simulink model "Energy_Cost"  (Simulink 8.8)
settings: Solver=ode23t  StartTime=0.0  StopTime=24  RelTol=1e-3  EnableMultiTasking=on
model workspace: external: MAT-File (data not in the file)
libraries: simulink x4
(part 3 of 5)

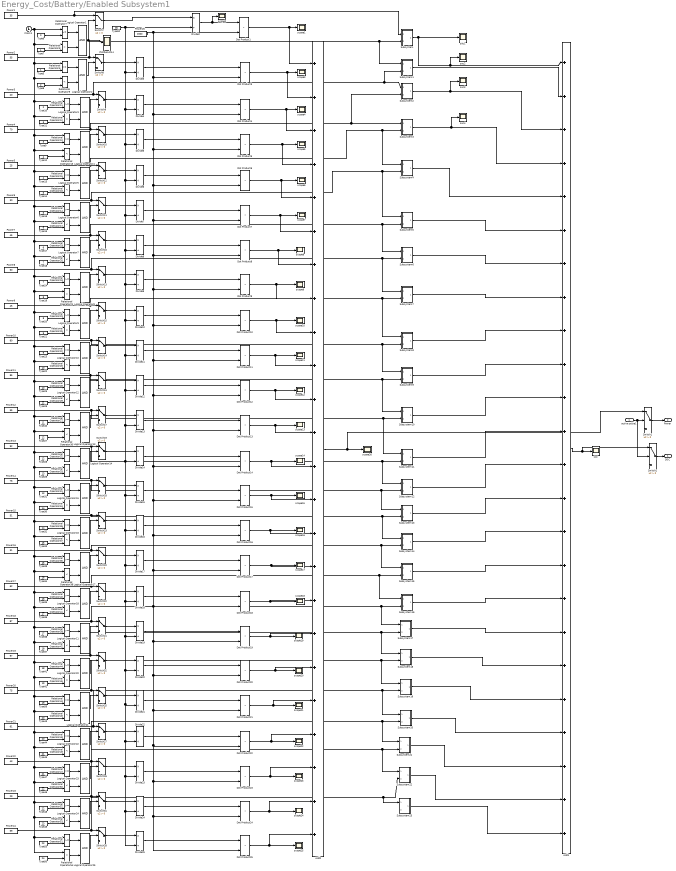
== system Energy_Cost/Battery/Enabled Subsystem1 ==
  active pulse1 : Inport
  Add1 : Sum  Inputs=++++++++++++++++++++++++
  Add2 : Sum  Inputs=++++++++++++++++++++++++
  Clock1 : Clock
  Divide{2..25} (24 alike) : Product  Inputs=*/
  Dot Product{1,3..25} (24 alike) : DotProduct  InputSameDT=on  OutDataTypeStr=Inherit: Inherit via internal rule
  Logical Operator{1..18,20..25} (24 alike) : Logic  AllPortsSameDT=off  OutDataTypeStr=boolean
  PlotResults4 : Scope
  Power1 : Constant  Value=35
  Power10 : Constant  Value=80
  Power11 : Constant  Value=85
  Power12 : Constant  Value=55
  Power13 : Constant  Value=92
  Power14 : Constant  Value=76
  Power15 : Constant  Value=51
  Power16 : Constant  Value=31
  Power17 : Constant  Value=62
  Power18 : Constant  Value=87
  Power19 : Constant  Value=97
  Power2 : Constant  Value=55
  Power20 : Constant  Value=75
  Power21 : Constant  Value=61
  Power22 : Constant  Value=43
  Power23 : Constant  Value=29
  Power24 : Constant  Value=59
  Power25 : Constant  Value=1500
  Power3 : Constant  Value=20
  Power4 : Constant  Value=70
  Power5 : Constant  Value=25
  Power6 : Constant  Value=30
  Power7 : Constant  Value=45
  Power8 : Constant  Value=60
  Power9 : Constant  Value=45
  Relational Operator{6..7,10..11,14..15,18..19,22..23,27..28,31..32,35..36,39..40,43..44,47..48,51..52} (24 alike) : RelationalOperator  RndMeth=Nearest  InputSameDT=on
  Relational Operator{8..9,12..13,16..17,20..21,25..26,29..30,33..34,37..38,41..42,45..46,49..50,53..54} (24 alike) : RelationalOperator  Operator=<  RndMeth=Nearest  InputSameDT=on
  Subsystem : Subsystem
  Subsystem1 : Subsystem
  Subsystem10 : Subsystem
  Subsystem11 : Subsystem
  Subsystem12 : Subsystem
  Subsystem13 : Subsystem
  Subsystem14 : Subsystem
  Subsystem15 : Subsystem
  Subsystem16 : Subsystem
  Subsystem17 : Subsystem
  Subsystem18 : Subsystem
  Subsystem19 : Subsystem
  Subsystem2 : Subsystem
  Subsystem20 : Subsystem
  Subsystem21 : Subsystem
  Subsystem22 : Subsystem
  Subsystem23 : Subsystem
  Subsystem3 : Subsystem
  Subsystem4 : Subsystem
  Subsystem5 : Subsystem
  Subsystem6 : Subsystem
  Subsystem7 : Subsystem
  Subsystem8 : Subsystem
  Subsystem9 : Subsystem
  Switch{1..2,7..28,31..32} (26 alike) : Switch  Criteria=u2 > Threshold
  Type10 : Constant  Value=2
  Type11 : Constant  Value=3
  Type12 : Constant  Value=4
  Type13 : Constant  Value=4
  Type14 : Constant  Value=5
  Type15 : Constant  Value=6
  Type16 : Constant  Value=5
  Type17 : Constant  Value=6
  Type18 : Constant  Value=7
  Type19 : Constant  Value=8
  Type20 : Constant  Value=8
  Type21 : Constant  Value=9
  Type22 : Constant  Value=10
  Type23 : Constant  Value=9
  Type24 : Constant  Value=7
  Type25 : Constant  Value=10
  Type26 : Constant  Value=11
  Type27 : Constant  Value=12
  Type28 : Constant  Value=12
  Type29 : Constant  Value=13
  Type30 : Constant  Value=14
  Type31 : Constant  Value=13
  Type32 : Constant  Value=14
  Type33 : Constant  Value=15
  Type34 : Constant  Value=16
  Type35 : Constant  Value=16
  Type36 : Constant  Value=17
  Type37 : Constant  Value=18
  Type38 : Constant  Value=17
  Type39 : Constant  Value=15
  Type40 : Constant  Value=11
  Type41 : Constant  Value=18
  Type42 : Constant  Value=19
  Type43 : Constant  Value=20
  Type44 : Constant  Value=20
  Type45 : Constant  Value=21
  Type46 : Constant  Value=22
  Type47 : Constant  Value=21
  Type48 : Constant  Value=22
  Type49 : Constant  Value=23
  Type5 : Constant
  Type50 : Constant  Value=24
  Type52 : Constant  Value=35
  Type55 : Constant  Value=23
  Type56 : Constant  Value=19
  Type6 : Constant  Value=0
  Type7 : Constant
  Type8 : Constant  Value=2
  Type9 : Constant  Value=3
  scope{1..26} (26 alike) : Scope
  soc{,1..4} (5 alike) : Scope
  SOC : Outport
  Power : Outport  Port=2
  wires:
  active pulse1/1 -> Switch1/2, Switch2/2
  Type36/1 -> Relational Operator41/2
  Relational Operator41/1 -> Logical Operator18/2
  Type38/1 -> Relational Operator39/2
  Type37/1 -> Relational Operator42/2
  Relational Operator42/1 -> Logical Operator11/2
  Relational Operator39/1 -> Logical Operator11/1
  Logical Operator11/1 -> Switch21/2
  Type41/1 -> Relational Operator44/2
  Type42/1 -> Relational Operator45/2
  Relational Operator45/1 -> Logical Operator20/2
  Relational Operator44/1 -> Logical Operator20/1
  Logical Operator20/1 -> Switch32/2
  Type56/1 -> Relational Operator43/2
  Type43/1 -> Relational Operator46/2
  Relational Operator46/1 -> Logical Operator21/2
  Relational Operator43/1 -> Logical Operator21/1
  Logical Operator21/1 -> Switch25/2
  Type44/1 -> Relational Operator48/2
  Type45/1 -> Relational Operator49/2
  Relational Operator49/1 -> Logical Operator22/2
  Relational Operator48/1 -> Logical Operator22/1
  Logical Operator22/1 -> Switch27/2
  Type47/1 -> Relational Operator47/2
  Type46/1 -> Relational Operator50/2
  Relational Operator50/1 -> Logical Operator23/2
  Relational Operator47/1 -> Logical Operator23/1
  Logical Operator23/1 -> Switch26/2
  Type48/1 -> Relational Operator52/2
  Type49/1 -> Relational Operator53/2
  Relational Operator53/1 -> Logical Operator24/2
  Relational Operator52/1 -> Logical Operator24/1
  Logical Operator24/1 -> Switch31/2
  Type55/1 -> Relational Operator51/2
  Type50/1 -> Relational Operator54/2
  Relational Operator54/1 -> Logical Operator25/2
  Relational Operator51/1 -> Logical Operator25/1
  Logical Operator25/1 -> Switch28/2
  Power18/1 -> Switch21/1, Subsystem16/2(In2), Subsystem17/1(In1)
  Power19/1 -> Switch32/1, Subsystem17/2(In2), Subsystem18/1(In1)
  Power20/1 -> Switch25/1, Subsystem18/2(In2), Subsystem19/1(In1)
  Power21/1 -> Switch27/1, Subsystem19/2(In2), Subsystem20/1(In1)
  Power22/1 -> Switch26/1, Subsystem20/2(In2), Subsystem21/1(In1)
  Power23/1 -> Switch31/1, Subsystem21/2(In2), Subsystem22/1(In1)
  Power24/1 -> Switch28/1, Subsystem22/2(In2), Subsystem23/1(In1)
  Power1/1 -> Switch7/1, Subsystem/1(In1)
  Switch7/1 -> Divide2/1
  Clock1/1 -> Relational Operator7/1, Relational Operator8/1, Relational Operator6/1, Relational Operator9/1, Relational Operator11/1, Relational Operator19/1, Relational Operator20/1, Relational Operator18/1, Relational Operator21/1, Relational Operator23/1, Relational Operator25/1, Relational Operator22/1, Relational Operator26/1, Relational Operator28/1, Relational Operator29/1, Relational Operator27/1, Relational Operator32/1, Relational Operator31/1, Relational Operator34/1, Relational Operator36/1, Relational Operator37/1, Relational Operator35/1, Relational Operator38/1, Relational Operator40/1, Relational Operator41/1, Relational Operator39/1, Relational Operator42/1, Relational Operator45/1, Relational Operator43/1, Relational Operator47/1, Relational Operator54/1, Relational Operator51/1, Relational Operator53/1, Relational Operator52/1, Relational Operator50/1, Relational Operator49/1, Relational Operator48/1, Relational Operator46/1, Relational Operator44/1, Relational Operator33/1, Relational Operator30/1, Relational Operator17/1, Relational Operator14/1, Relational Operator16/1, Relational Operator15/1, Relational Operator13/1, Relational Operator10/1, Relational Operator12/1
  Type6/1 -> Relational Operator7/2
  Relational Operator7/1 -> Logical Operator1/1
  Power2/1 -> Switch8/1, Subsystem/2(In2), Subsystem1/1(In1)
  Type5/1 -> Relational Operator6/2
  Relational Operator6/1 -> Logical Operator2/1
  Type10/1 -> Relational Operator11/2
  Relational Operator11/1 -> Logical Operator3/1
  Type9/1 -> Relational Operator10/2
  Type12/1 -> Relational Operator13/2
  Relational Operator13/1 -> Logical Operator4/2
  Relational Operator10/1 -> Logical Operator4/1
  Logical Operator4/1 -> Switch10/2
  Type13/1 -> Relational Operator15/2
  Type14/1 -> Relational Operator16/2
  Relational Operator16/1 -> Logical Operator5/2
  Relational Operator15/1 -> Logical Operator5/1
  Logical Operator5/1 -> Switch12/2
  Type16/1 -> Relational Operator14/2
  Type15/1 -> Relational Operator17/2
  Relational Operator17/1 -> Logical Operator6/2
  Relational Operator14/1 -> Logical Operator6/1
  Logical Operator6/1 -> Switch11/2
  Type17/1 -> Relational Operator19/2
  Type18/1 -> Relational Operator20/2
  Relational Operator20/1 -> Logical Operator7/2
  Relational Operator19/1 -> Logical Operator7/1
  Logical Operator7/1 -> Switch16/2
  Type24/1 -> Relational Operator18/2
  Type19/1 -> Relational Operator21/2
  Relational Operator21/1 -> Logical Operator8/2
  Relational Operator18/1 -> Logical Operator8/1
  Logical Operator8/1 -> Switch13/2
  Type20/1 -> Relational Operator23/2
  Type21/1 -> Relational Operator25/2
  Relational Operator25/1 -> Logical Operator9/2
  Relational Operator23/1 -> Logical Operator9/1
  Logical Operator9/1 -> Switch15/2
  Type23/1 -> Relational Operator22/2
  Type22/1 -> Relational Operator26/2
  Relational Operator26/1 -> Logical Operator10/2
  Relational Operator22/1 -> Logical Operator10/1
  Logical Operator10/1 -> Switch14/2
  Type25/1 -> Relational Operator28/2
  Type26/1 -> Relational Operator29/2
  Relational Operator29/1 -> Logical Operator12/2
  Relational Operator28/1 -> Logical Operator12/1
  Logical Operator12/1 -> Switch24/2
  Type40/1 -> Relational Operator27/2
  Type27/1 -> Relational Operator30/2
  Relational Operator30/1 -> Logical Operator13/2
  Relational Operator27/1 -> Logical Operator13/1
  Logical Operator13/1 -> Switch17/2
  Type28/1 -> Relational Operator32/2
  Type29/1 -> Relational Operator33/2
  Relational Operator33/1 -> Logical Operator14/2
  Relational Operator32/1 -> Logical Operator14/1
  Logical Operator14/1 -> Switch19/2
  Type31/1 -> Relational Operator31/2
  Type30/1 -> Relational Operator34/2
  Relational Operator34/1 -> Logical Operator15/2
  Relational Operator31/1 -> Logical Operator15/1
  Logical Operator15/1 -> Switch18/2
  Type32/1 -> Relational Operator36/2
  Type33/1 -> Relational Operator37/2
  Relational Operator37/1 -> Logical Operator16/2
  Relational Operator36/1 -> Logical Operator16/1
  Logical Operator16/1 -> Switch23/2
  Type39/1 -> Relational Operator35/2
  Type34/1 -> Relational Operator38/2
  Relational Operator38/1 -> Logical Operator17/2
  Relational Operator35/1 -> Logical Operator17/1
  Logical Operator17/1 -> Switch20/2
  Type35/1 -> Relational Operator40/2
  Relational Operator40/1 -> Logical Operator18/1
  Logical Operator18/1 -> Switch22/2
  Power3/1 -> Switch9/1, Subsystem1/2(In2), Subsystem2/1(In1)
  Power4/1 -> Switch10/1, Subsystem2/2(In2), Subsystem3/1(In1)
  Power5/1 -> Switch12/1, Subsystem3/2(In2), Subsystem4/1(In1)
  Power6/1 -> Switch11/1, Subsystem4/2(In2), Subsystem5/1(In1)
  Power7/1 -> Switch16/1, Subsystem5/2(In2), Subsystem6/1(In1)
  Power8/1 -> Switch13/1, Subsystem6/2(In2), Subsystem7/1(In1)
  Power9/1 -> Switch15/1, Subsystem7/2(In2), Subsystem8/1(In1)
  Power10/1 -> Switch14/1, Subsystem8/2(In2), Subsystem9/1(In1)
  Power11/1 -> Switch24/1, Subsystem9/2(In2), Subsystem10/1(In1)
  Power12/1 -> Switch17/1, Subsystem10/2(In2), Subsystem11/1(In1)
  Power13/1 -> Switch19/1, Subsystem11/2(In2), Subsystem12/1(In1)
  Power14/1 -> Switch18/1, Subsystem12/2(In2), Subsystem13/1(In1)
  Power15/1 -> Switch23/1, Subsystem13/2(In2), Subsystem14/1(In1)
  Power16/1 -> Switch20/1, Subsystem14/2(In2), Subsystem15/1(In1)
  Power17/1 -> Switch22/1, Subsystem15/2(In2), Subsystem16/1(In1)
  Type52/1 -> Divide2/2, Divide3/2, Divide4/2, Divide5/2, Divide9/2, Divide10/2, Divide12/2, Divide13/2, Divide18/2, Divide19/2, Divide20/2, Divide21/2, Divide22/2, Divide23/2, Divide25/2, Divide24/2, Divide17/2, Divide16/2, Divide15/2, Divide14/2, Divide11/2, Divide8/2, Divide7/2, Divide6/2
  Divide2/1 -> Dot Product1/1, scope2/1
  Power25/1 -> Dot Product1/2, Dot Product3/2, Dot Product4/2, Dot Product6/2, Dot Product7/2, Dot Product12/2, Dot Product13/2, Dot Product14/2, Dot Product18/2, Dot Product19/2, Dot Product20/2, Dot Product21/2, Dot Product22/2, Dot Product23/2, Dot Product25/2, Dot Product24/2, Dot Product17/2, Dot Product16/2, Dot Product15/2, Dot Product11/2, Dot Product10/2, Dot Product9/2, Dot Product8/2, Dot Product5/2
  Dot Product1/1 -> scope1/1, Add2/1
  Switch8/1 -> Divide3/1
  Divide3/1 -> Dot Product3/1
  Dot Product3/1 -> scope3/1, Add2/2
  Divide4/1 -> Dot Product4/1
  Dot Product4/1 -> scope4/1, Add2/3
  Divide5/1 -> Dot Product5/1
  Dot Product5/1 -> scope5/1, Add2/4
  Divide6/1 -> Dot Product6/1
  Dot Product6/1 -> scope6/1, Add2/5
  Divide7/1 -> Dot Product7/1
  Dot Product7/1 -> scope7/1, Add2/6
  Divide8/1 -> Dot Product8/1
  Dot Product8/1 -> scope8/1, Add2/7
  Divide9/1 -> Dot Product9/1
  Dot Product9/1 -> scope9/1, Add2/8
  Divide10/1 -> Dot Product10/1
  Dot Product10/1 -> scope10/1, Add2/9
  Divide11/1 -> Dot Product11/1
  Dot Product11/1 -> scope11/1, Add2/10
  Divide12/1 -> Dot Product12/1
  Dot Product12/1 -> scope12/1, Add2/11
  Divide13/1 -> Dot Product13/1
  Dot Product13/1 -> scope13/1, Add2/12
  Divide14/1 -> Dot Product14/1
  Dot Product14/1 -> scope14/1, Add2/13
  Divide15/1 -> Dot Product15/1
  Dot Product15/1 -> scope15/1, Add2/14
  Divide16/1 -> Dot Product16/1
  Dot Product16/1 -> scope16/1, Add2/15
  Divide17/1 -> Dot Product17/1
  Dot Product17/1 -> scope17/1, Add2/16
  Divide18/1 -> Dot Product18/1
  Dot Product18/1 -> scope18/1, Add2/17
  Divide19/1 -> Dot Product19/1
  Dot Product19/1 -> scope19/1, Add2/18
  Divide20/1 -> Dot Product20/1
  Dot Product20/1 -> scope20/1, Add2/19
  Divide21/1 -> Dot Product21/1
  Dot Product21/1 -> scope21/1, Add2/20
  Divide22/1 -> Dot Product22/1
  Dot Product22/1 -> scope22/1, Add2/21
  Divide23/1 -> Dot Product23/1
  Dot Product23/1 -> scope23/1, Add2/22
  Divide24/1 -> Dot Product24/1
  Dot Product24/1 -> scope24/1, Add2/23
  Divide25/1 -> Dot Product25/1
  Dot Product25/1 -> scope25/1, Add2/24
  Switch28/1 -> Divide25/1
  Switch31/1 -> Divide24/1
  Switch26/1 -> Divide23/1
  Switch27/1 -> Divide22/1
  Switch25/1 -> Divide21/1
  Switch32/1 -> Divide20/1
  Switch21/1 -> Divide19/1
  Switch22/1 -> Divide18/1
  Switch20/1 -> Divide17/1
  Switch23/1 -> Divide16/1
  Switch18/1 -> Divide15/1
  Switch19/1 -> Divide14/1
  Switch17/1 -> Divide13/1
  Switch24/1 -> Divide12/1
  Switch14/1 -> Divide11/1
  Switch15/1 -> Divide10/1
  Switch13/1 -> Divide9/1
  Switch16/1 -> Divide8/1
  Switch11/1 -> Divide7/1
  Switch12/1 -> Divide6/1
  Switch10/1 -> Divide5/1
  Switch9/1 -> Divide4/1
  Add2/1 -> scope26/1, Switch1/1
  Logical Operator3/1 -> Switch9/2
  Relational Operator12/1 -> Logical Operator3/2
  Type11/1 -> Relational Operator12/2
  Logical Operator2/1 -> Switch8/2
  Type8/1 -> Relational Operator9/2
  Relational Operator9/1 -> Logical Operator2/2
  Logical Operator1/1 -> Switch7/2, PlotResults4/1
  Type7/1 -> Relational Operator8/2
  Relational Operator8/1 -> Logical Operator1/2
  Subsystem/1(Out1) -> soc1/1, Add1/1, soc2/1
  Subsystem1/1(Out1) -> Add1/2
  Subsystem2/1(Out1) -> soc3/1, Add1/3
  Subsystem3/1(Out1) -> Add1/4, soc4/1
  Add1/1 -> soc/1, Switch2/1
  Subsystem4/1(Out1) -> Add1/5
  Subsystem5/1(Out1) -> Add1/6
  Subsystem6/1(Out1) -> Add1/7
  Subsystem7/1(Out1) -> Add1/8
  Subsystem8/1(Out1) -> Add1/9
  Subsystem9/1(Out1) -> Add1/10
  Subsystem10/1(Out1) -> Add1/11
  Subsystem11/1(Out1) -> Add1/12
  Subsystem12/1(Out1) -> Add1/13
  Subsystem13/1(Out1) -> Add1/14
  Subsystem14/1(Out1) -> Add1/15
  Subsystem15/1(Out1) -> Add1/16
  Subsystem16/1(Out1) -> Add1/17
  Subsystem17/1(Out1) -> Add1/18
  Subsystem18/1(Out1) -> Add1/19
  Subsystem19/1(Out1) -> Add1/20
  Subsystem20/1(Out1) -> Add1/21
  Subsystem21/1(Out1) -> Add1/22
  Subsystem22/1(Out1) -> Add1/23
  Subsystem23/1(Out1) -> Add1/24
  Switch2/1 -> SOC/1
  Switch1/1 -> Power/1

== system Energy_Cost/Battery/Rates ==
  Powe_cons : Inport
  Rate_season : Inport  Port=2
  Clock1 : Clock
      settings: Decimation=100
  Constant : Constant  Value=6.2
  Constant1 : Constant  Value=10.8
  Constant2 : Constant  Value=9.2
  Electricity Rate : M-S-Function  FunctionName=Elec_Rate_Fun
  Heater Switch1 : Product  RndMeth=Zero
  Rate : Outport  InitialOutput=0
  wires:
  Rate_season/1 -> Electricity Rate/5
  Clock1/1 -> Electricity Rate/4
  Constant/1 -> Electricity Rate/1
  Heater Switch1/1 -> Rate/1
  Powe_cons/1 -> Heater Switch1/2
  Electricity Rate/1 -> Heater Switch1/1  "Elec_Rate"
  Constant1/1 -> Electricity Rate/3
  Constant2/1 -> Electricity Rate/2

== system Energy_Cost/Battery/Subsystem ==
  In1 : Inport
  In2 : Inport  Port=2
  Clock2 : Clock
  Divide26 : Product  Inputs=*/
  Dot Product2 : DotProduct  InputSameDT=on  OutDataTypeStr=Inherit: Inherit via internal rule
  Logical Operator19 : Logic  AllPortsSameDT=off  OutDataTypeStr=boolean
  Relational Operator2 : RelationalOperator  RndMeth=Nearest  InputSameDT=on
  Relational Operator3 : RelationalOperator  Operator=<  RndMeth=Nearest  InputSameDT=on
  Sum : Sum  Inputs=|++
  Sum1 : Sum  Inputs=|-+
  Switch2 : Switch  Criteria=u2 > Threshold
  Type54 : Constant
  Type57 : Constant  Value=0
  Type58 : Constant
  soc3 : Scope
  Out1 : Outport
  wires:
  Sum1/1 -> Divide26/1
  Type54/1 -> Divide26/2
  Divide26/1 -> Dot Product2/1
  Clock2/1 -> Dot Product2/2, Relational Operator3/1, Relational Operator2/1
  Dot Product2/1 -> Sum/2
  Sum/1 -> Switch2/1
  Type57/1 -> Relational Operator2/2
  Relational Operator2/1 -> Logical Operator19/1
  Type58/1 -> Relational Operator3/2
  Relational Operator3/1 -> Logical Operator19/2
  Logical Operator19/1 -> Switch2/2
  In1/1 -> Sum/1, Sum1/1
  In2/1 -> Sum1/2
  Switch2/1 -> Out1/1, soc3/1

== system Energy_Cost/Battery/Subsystem1 ==
  In1 : Inport
  In2 : Inport  Port=2
  Clock2 : Clock
  Divide26 : Product  Inputs=*/
  Dot Product2 : DotProduct  InputSameDT=on  OutDataTypeStr=Inherit: Inherit via internal rule
  Logical Operator19 : Logic  AllPortsSameDT=off  OutDataTypeStr=boolean
  Relational Operator2 : RelationalOperator  RndMeth=Nearest  InputSameDT=on
  Relational Operator3 : RelationalOperator  Operator=<  RndMeth=Nearest  InputSameDT=on
  Sum : Sum  Inputs=|++
  Sum1 : Sum  Inputs=|-+
  Sum2 : Sum  Inputs=|+-
  Switch2 : Switch  Criteria=u2 > Threshold
  Type1 : Constant
  Type54 : Constant
  Type57 : Constant
  Type58 : Constant  Value=2
  soc1 : Scope
  Out1 : Outport
  wires:
  Switch2/1 -> Out1/1, soc1/1
  In2/1 -> Sum1/2
  In1/1 -> Sum1/1, Sum/1
  Logical Operator19/1 -> Switch2/2
  Relational Operator3/1 -> Logical Operator19/2
  Type58/1 -> Relational Operator3/2
  Relational Operator2/1 -> Logical Operator19/1
  Type57/1 -> Relational Operator2/2
  Sum/1 -> Switch2/1
  Dot Product2/1 -> Sum/2
  Divide26/1 -> Dot Product2/1
  Type54/1 -> Divide26/2
  Sum1/1 -> Divide26/1
  Clock2/1 -> Sum2/1, Relational Operator2/1, Relational Operator3/1
  Type1/1 -> Sum2/2
  Sum2/1 -> Dot Product2/2

== system Energy_Cost/Battery/Subsystem10 ==
  In1 : Inport
  In2 : Inport  Port=2
  Clock2 : Clock
  Divide26 : Product  Inputs=*/
  Dot Product2 : DotProduct  InputSameDT=on  OutDataTypeStr=Inherit: Inherit via internal rule
  Logical Operator19 : Logic  AllPortsSameDT=off  OutDataTypeStr=boolean
  Relational Operator2 : RelationalOperator  RndMeth=Nearest  InputSameDT=on
  Relational Operator3 : RelationalOperator  Operator=<  RndMeth=Nearest  InputSameDT=on
  Sum : Sum  Inputs=|++
  Sum1 : Sum  Inputs=|-+
  Sum2 : Sum  Inputs=|+-
  Switch2 : Switch  Criteria=u2 > Threshold
  Type1 : Constant  Value=10
  Type54 : Constant
  Type57 : Constant  Value=10
  Type58 : Constant  Value=11
  soc1 : Scope
  Out1 : Outport
  wires:
  Sum2/1 -> Dot Product2/2
  Type1/1 -> Sum2/2
  Clock2/1 -> Relational Operator3/1, Relational Operator2/1, Sum2/1
  Sum1/1 -> Divide26/1
  Type54/1 -> Divide26/2
  Divide26/1 -> Dot Product2/1
  Dot Product2/1 -> Sum/2
  Sum/1 -> Switch2/1
  Type57/1 -> Relational Operator2/2
  Relational Operator2/1 -> Logical Operator19/1
  Type58/1 -> Relational Operator3/2
  Relational Operator3/1 -> Logical Operator19/2
  Logical Operator19/1 -> Switch2/2
  In1/1 -> Sum/1, Sum1/1
  In2/1 -> Sum1/2
  Switch2/1 -> soc1/1, Out1/1

== system Energy_Cost/Battery/Subsystem11 ==
  In1 : Inport
  In2 : Inport  Port=2
  Clock2 : Clock
  Divide26 : Product  Inputs=*/
  Dot Product2 : DotProduct  InputSameDT=on  OutDataTypeStr=Inherit: Inherit via internal rule
  Logical Operator19 : Logic  AllPortsSameDT=off  OutDataTypeStr=boolean
  Relational Operator2 : RelationalOperator  RndMeth=Nearest  InputSameDT=on
  Relational Operator3 : RelationalOperator  Operator=<  RndMeth=Nearest  InputSameDT=on
  Sum : Sum  Inputs=|++
  Sum1 : Sum  Inputs=|-+
  Sum2 : Sum  Inputs=|+-
  Switch2 : Switch  Criteria=u2 > Threshold
  Type1 : Constant  Value=11
  Type54 : Constant
  Type57 : Constant  Value=11
  Type58 : Constant  Value=12
  soc1 : Scope
  Out1 : Outport
  wires:
  Switch2/1 -> Out1/1, soc1/1
  In2/1 -> Sum1/2
  In1/1 -> Sum1/1, Sum/1
  Logical Operator19/1 -> Switch2/2
  Relational Operator3/1 -> Logical Operator19/2
  Type58/1 -> Relational Operator3/2
  Relational Operator2/1 -> Logical Operator19/1
  Type57/1 -> Relational Operator2/2
  Sum/1 -> Switch2/1
  Dot Product2/1 -> Sum/2
  Divide26/1 -> Dot Product2/1
  Type54/1 -> Divide26/2
  Sum1/1 -> Divide26/1
  Clock2/1 -> Sum2/1, Relational Operator2/1, Relational Operator3/1
  Type1/1 -> Sum2/2
  Sum2/1 -> Dot Product2/2

== system Energy_Cost/Battery/Subsystem12 ==
  In1 : Inport
  In2 : Inport  Port=2
  Clock2 : Clock
  Divide26 : Product  Inputs=*/
  Dot Product2 : DotProduct  InputSameDT=on  OutDataTypeStr=Inherit: Inherit via internal rule
  Logical Operator19 : Logic  AllPortsSameDT=off  OutDataTypeStr=boolean
  Relational Operator2 : RelationalOperator  RndMeth=Nearest  InputSameDT=on
  Relational Operator3 : RelationalOperator  Operator=<  RndMeth=Nearest  InputSameDT=on
  Sum : Sum  Inputs=|++
  Sum1 : Sum  Inputs=|-+
  Sum2 : Sum  Inputs=|+-
  Switch2 : Switch  Criteria=u2 > Threshold
  Type1 : Constant  Value=12
  Type54 : Constant
  Type57 : Constant  Value=12
  Type58 : Constant  Value=13
  soc1 : Scope
  Out1 : Outport
  wires:
  Sum2/1 -> Dot Product2/2
  Type1/1 -> Sum2/2
  Clock2/1 -> Relational Operator3/1, Relational Operator2/1, Sum2/1
  Sum1/1 -> Divide26/1
  Type54/1 -> Divide26/2
  Divide26/1 -> Dot Product2/1
  Dot Product2/1 -> Sum/2
  Sum/1 -> Switch2/1
  Type57/1 -> Relational Operator2/2
  Relational Operator2/1 -> Logical Operator19/1
  Type58/1 -> Relational Operator3/2
  Relational Operator3/1 -> Logical Operator19/2
  Logical Operator19/1 -> Switch2/2
  In1/1 -> Sum/1, Sum1/1
  In2/1 -> Sum1/2
  Switch2/1 -> soc1/1, Out1/1

== system Energy_Cost/Battery/Subsystem13 ==
  In1 : Inport
  In2 : Inport  Port=2
  Clock2 : Clock
  Divide26 : Product  Inputs=*/
  Dot Product2 : DotProduct  InputSameDT=on  OutDataTypeStr=Inherit: Inherit via internal rule
  Logical Operator19 : Logic  AllPortsSameDT=off  OutDataTypeStr=boolean
  Relational Operator2 : RelationalOperator  RndMeth=Nearest  InputSameDT=on
  Relational Operator3 : RelationalOperator  Operator=<  RndMeth=Nearest  InputSameDT=on
  Sum : Sum  Inputs=|++
  Sum1 : Sum  Inputs=|-+
  Sum2 : Sum  Inputs=|+-
  Switch2 : Switch  Criteria=u2 > Threshold
  Type1 : Constant  Value=13
  Type54 : Constant
  Type57 : Constant  Value=13
  Type58 : Constant  Value=14
  soc1 : Scope
  Out1 : Outport
  wires:
  Switch2/1 -> Out1/1, soc1/1
  In2/1 -> Sum1/2
  In1/1 -> Sum1/1, Sum/1
  Logical Operator19/1 -> Switch2/2
  Relational Operator3/1 -> Logical Operator19/2
  Type58/1 -> Relational Operator3/2
  Relational Operator2/1 -> Logical Operator19/1
  Type57/1 -> Relational Operator2/2
  Sum/1 -> Switch2/1
  Dot Product2/1 -> Sum/2
  Divide26/1 -> Dot Product2/1
  Type54/1 -> Divide26/2
  Sum1/1 -> Divide26/1
  Clock2/1 -> Sum2/1, Relational Operator2/1, Relational Operator3/1
  Type1/1 -> Sum2/2
  Sum2/1 -> Dot Product2/2

== system Energy_Cost/Battery/Subsystem14 ==
  In1 : Inport
  In2 : Inport  Port=2
  Clock2 : Clock
  Divide26 : Product  Inputs=*/
  Dot Product2 : DotProduct  InputSameDT=on  OutDataTypeStr=Inherit: Inherit via internal rule
  Logical Operator19 : Logic  AllPortsSameDT=off  OutDataTypeStr=boolean
  Relational Operator2 : RelationalOperator  RndMeth=Nearest  InputSameDT=on
  Relational Operator3 : RelationalOperator  Operator=<  RndMeth=Nearest  InputSameDT=on
  Sum : Sum  Inputs=|++
  Sum1 : Sum  Inputs=|-+
  Sum2 : Sum  Inputs=|+-
  Switch2 : Switch  Criteria=u2 > Threshold
  Type1 : Constant  Value=14
  Type54 : Constant
  Type57 : Constant  Value=14
  Type58 : Constant  Value=15
  soc1 : Scope
  Out1 : Outport
  wires:
  Sum2/1 -> Dot Product2/2
  Type1/1 -> Sum2/2
  Clock2/1 -> Relational Operator3/1, Relational Operator2/1, Sum2/1
  Sum1/1 -> Divide26/1
  Type54/1 -> Divide26/2
  Divide26/1 -> Dot Product2/1
  Dot Product2/1 -> Sum/2
  Sum/1 -> Switch2/1
  Type57/1 -> Relational Operator2/2
  Relational Operator2/1 -> Logical Operator19/1
  Type58/1 -> Relational Operator3/2
  Relational Operator3/1 -> Logical Operator19/2
  Logical Operator19/1 -> Switch2/2
  In1/1 -> Sum/1, Sum1/1
  In2/1 -> Sum1/2
  Switch2/1 -> soc1/1, Out1/1

== system Energy_Cost/Battery/Subsystem15 ==
  In1 : Inport
  In2 : Inport  Port=2
  Clock2 : Clock
  Divide26 : Product  Inputs=*/
  Dot Product2 : DotProduct  InputSameDT=on  OutDataTypeStr=Inherit: Inherit via internal rule
  Logical Operator19 : Logic  AllPortsSameDT=off  OutDataTypeStr=boolean
  Relational Operator2 : RelationalOperator  RndMeth=Nearest  InputSameDT=on
  Relational Operator3 : RelationalOperator  Operator=<  RndMeth=Nearest  InputSameDT=on
  Sum : Sum  Inputs=|++
  Sum1 : Sum  Inputs=|-+
  Sum2 : Sum  Inputs=|+-
  Switch2 : Switch  Criteria=u2 > Threshold
  Type1 : Constant  Value=15
  Type54 : Constant
  Type57 : Constant  Value=15
  Type58 : Constant  Value=16
  soc1 : Scope
  Out1 : Outport
  wires:
  Switch2/1 -> Out1/1, soc1/1
  In2/1 -> Sum1/2
  In1/1 -> Sum1/1, Sum/1
  Logical Operator19/1 -> Switch2/2
  Relational Operator3/1 -> Logical Operator19/2
  Type58/1 -> Relational Operator3/2
  Relational Operator2/1 -> Logical Operator19/1
  Type57/1 -> Relational Operator2/2
  Sum/1 -> Switch2/1
  Dot Product2/1 -> Sum/2
  Divide26/1 -> Dot Product2/1
  Type54/1 -> Divide26/2
  Sum1/1 -> Divide26/1
  Clock2/1 -> Sum2/1, Relational Operator2/1, Relational Operator3/1
  Type1/1 -> Sum2/2
  Sum2/1 -> Dot Product2/2

== system Energy_Cost/Battery/Subsystem16 ==
  In1 : Inport
  In2 : Inport  Port=2
  Clock2 : Clock
  Divide26 : Product  Inputs=*/
  Dot Product2 : DotProduct  InputSameDT=on  OutDataTypeStr=Inherit: Inherit via internal rule
  Logical Operator19 : Logic  AllPortsSameDT=off  OutDataTypeStr=boolean
  Relational Operator2 : RelationalOperator  RndMeth=Nearest  InputSameDT=on
  Relational Operator3 : RelationalOperator  Operator=<  RndMeth=Nearest  InputSameDT=on
  Sum : Sum  Inputs=|++
  Sum1 : Sum  Inputs=|-+
  Sum2 : Sum  Inputs=|+-
  Switch2 : Switch  Criteria=u2 > Threshold
  Type1 : Constant  Value=16
  Type54 : Constant
  Type57 : Constant  Value=16
  Type58 : Constant  Value=17
  soc1 : Scope
  Out1 : Outport
  wires:
  Sum2/1 -> Dot Product2/2
  Type1/1 -> Sum2/2
  Clock2/1 -> Relational Operator3/1, Relational Operator2/1, Sum2/1
  Sum1/1 -> Divide26/1
  Type54/1 -> Divide26/2
  Divide26/1 -> Dot Product2/1
  Dot Product2/1 -> Sum/2
  Sum/1 -> Switch2/1
  Type57/1 -> Relational Operator2/2
  Relational Operator2/1 -> Logical Operator19/1
  Type58/1 -> Relational Operator3/2
  Relational Operator3/1 -> Logical Operator19/2
  Logical Operator19/1 -> Switch2/2
  In1/1 -> Sum/1, Sum1/1
  In2/1 -> Sum1/2
  Switch2/1 -> soc1/1, Out1/1

== system Energy_Cost/Battery/Subsystem17 ==
  In1 : Inport
  In2 : Inport  Port=2
  Clock2 : Clock
  Divide26 : Product  Inputs=*/
  Dot Product2 : DotProduct  InputSameDT=on  OutDataTypeStr=Inherit: Inherit via internal rule
  Logical Operator19 : Logic  AllPortsSameDT=off  OutDataTypeStr=boolean
  Relational Operator2 : RelationalOperator  RndMeth=Nearest  InputSameDT=on
  Relational Operator3 : RelationalOperator  Operator=<  RndMeth=Nearest  InputSameDT=on
  Sum : Sum  Inputs=|++
  Sum1 : Sum  Inputs=|-+
  Sum2 : Sum  Inputs=|+-
  Switch2 : Switch  Criteria=u2 > Threshold
  Type1 : Constant  Value=17
  Type54 : Constant
  Type57 : Constant  Value=17
  Type58 : Constant  Value=18
  soc1 : Scope
  Out1 : Outport
  wires:
  Sum2/1 -> Dot Product2/2
  Type1/1 -> Sum2/2
  Clock2/1 -> Relational Operator3/1, Relational Operator2/1, Sum2/1
  Sum1/1 -> Divide26/1
  Type54/1 -> Divide26/2
  Divide26/1 -> Dot Product2/1
  Dot Product2/1 -> Sum/2
  Sum/1 -> Switch2/1
  Type57/1 -> Relational Operator2/2
  Relational Operator2/1 -> Logical Operator19/1
  Type58/1 -> Relational Operator3/2
  Relational Operator3/1 -> Logical Operator19/2
  Logical Operator19/1 -> Switch2/2
  In1/1 -> Sum/1, Sum1/1
  In2/1 -> Sum1/2
  Switch2/1 -> soc1/1, Out1/1

== system Energy_Cost/Battery/Subsystem18 ==
  In1 : Inport
  In2 : Inport  Port=2
  Clock2 : Clock
  Divide26 : Product  Inputs=*/
  Dot Product2 : DotProduct  InputSameDT=on  OutDataTypeStr=Inherit: Inherit via internal rule
  Logical Operator19 : Logic  AllPortsSameDT=off  OutDataTypeStr=boolean
  Relational Operator2 : RelationalOperator  RndMeth=Nearest  InputSameDT=on
  Relational Operator3 : RelationalOperator  Operator=<  RndMeth=Nearest  InputSameDT=on
  Sum : Sum  Inputs=|++
  Sum1 : Sum  Inputs=|-+
  Sum2 : Sum  Inputs=|+-
  Switch2 : Switch  Criteria=u2 > Threshold
  Type1 : Constant  Value=18
  Type54 : Constant
  Type57 : Constant  Value=18
  Type58 : Constant  Value=19
  soc1 : Scope
  Out1 : Outport
  wires:
  Switch2/1 -> Out1/1, soc1/1
  In2/1 -> Sum1/2
  In1/1 -> Sum1/1, Sum/1
  Logical Operator19/1 -> Switch2/2
  Relational Operator3/1 -> Logical Operator19/2
  Type58/1 -> Relational Operator3/2
  Relational Operator2/1 -> Logical Operator19/1
  Type57/1 -> Relational Operator2/2
  Sum/1 -> Switch2/1
  Dot Product2/1 -> Sum/2
  Divide26/1 -> Dot Product2/1
  Type54/1 -> Divide26/2
  Sum1/1 -> Divide26/1
  Clock2/1 -> Sum2/1, Relational Operator2/1, Relational Operator3/1
  Type1/1 -> Sum2/2
  Sum2/1 -> Dot Product2/2

== system Energy_Cost/Battery/Subsystem19 ==
  In1 : Inport
  In2 : Inport  Port=2
  Clock2 : Clock
  Divide26 : Product  Inputs=*/
  Dot Product2 : DotProduct  InputSameDT=on  OutDataTypeStr=Inherit: Inherit via internal rule
  Logical Operator19 : Logic  AllPortsSameDT=off  OutDataTypeStr=boolean
  Relational Operator2 : RelationalOperator  RndMeth=Nearest  InputSameDT=on
  Relational Operator3 : RelationalOperator  Operator=<  RndMeth=Nearest  InputSameDT=on
  Sum : Sum  Inputs=|++
  Sum1 : Sum  Inputs=|-+
  Sum2 : Sum  Inputs=|+-
  Switch2 : Switch  Criteria=u2 > Threshold
  Type1 : Constant  Value=19
  Type54 : Constant
  Type57 : Constant  Value=19
  Type58 : Constant  Value=20
  soc1 : Scope
  Out1 : Outport
  wires:
  Sum2/1 -> Dot Product2/2
  Type1/1 -> Sum2/2
  Clock2/1 -> Relational Operator3/1, Relational Operator2/1, Sum2/1
  Sum1/1 -> Divide26/1
  Type54/1 -> Divide26/2
  Divide26/1 -> Dot Product2/1
  Dot Product2/1 -> Sum/2
  Sum/1 -> Switch2/1
  Type57/1 -> Relational Operator2/2
  Relational Operator2/1 -> Logical Operator19/1
  Type58/1 -> Relational Operator3/2
  Relational Operator3/1 -> Logical Operator19/2
  Logical Operator19/1 -> Switch2/2
  In1/1 -> Sum/1, Sum1/1
  In2/1 -> Sum1/2
  Switch2/1 -> soc1/1, Out1/1

== system Energy_Cost/Battery/Subsystem2 ==
  In1 : Inport
  In2 : Inport  Port=2
  Clock2 : Clock
  Divide26 : Product  Inputs=*/
  Dot Product2 : DotProduct  InputSameDT=on  OutDataTypeStr=Inherit: Inherit via internal rule
  Logical Operator19 : Logic  AllPortsSameDT=off  OutDataTypeStr=boolean
  Relational Operator2 : RelationalOperator  RndMeth=Nearest  InputSameDT=on
  Relational Operator3 : RelationalOperator  Operator=<  RndMeth=Nearest  InputSameDT=on
  Sum : Sum  Inputs=|++
  Sum1 : Sum  Inputs=|-+
  Sum2 : Sum  Inputs=|+-
  Switch2 : Switch  Criteria=u2 > Threshold
  Type1 : Constant  Value=2
  Type54 : Constant
  Type57 : Constant  Value=2
  Type58 : Constant  Value=3
  soc1 : Scope
  Out1 : Outport
  wires:
  Sum2/1 -> Dot Product2/2
  Type1/1 -> Sum2/2
  Clock2/1 -> Relational Operator3/1, Relational Operator2/1, Sum2/1
  Sum1/1 -> Divide26/1
  Type54/1 -> Divide26/2
  Divide26/1 -> Dot Product2/1
  Dot Product2/1 -> Sum/2
  Sum/1 -> Switch2/1
  Type57/1 -> Relational Operator2/2
  Relational Operator2/1 -> Logical Operator19/1
  Type58/1 -> Relational Operator3/2
  Relational Operator3/1 -> Logical Operator19/2
  Logical Operator19/1 -> Switch2/2
  In1/1 -> Sum/1, Sum1/1
  In2/1 -> Sum1/2
  Switch2/1 -> soc1/1, Out1/1

== system Energy_Cost/Battery/Subsystem20 ==
  In1 : Inport
  In2 : Inport  Port=2
  Clock2 : Clock
  Divide26 : Product  Inputs=*/
  Dot Product2 : DotProduct  InputSameDT=on  OutDataTypeStr=Inherit: Inherit via internal rule
  Logical Operator19 : Logic  AllPortsSameDT=off  OutDataTypeStr=boolean
  Relational Operator2 : RelationalOperator  RndMeth=Nearest  InputSameDT=on
  Relational Operator3 : RelationalOperator  Operator=<  RndMeth=Nearest  InputSameDT=on
  Sum : Sum  Inputs=|++
  Sum1 : Sum  Inputs=|-+
  Sum2 : Sum  Inputs=|+-
  Switch2 : Switch  Criteria=u2 > Threshold
  Type1 : Constant  Value=20
  Type54 : Constant
  Type57 : Constant  Value=20
  Type58 : Constant  Value=21
  soc1 : Scope
  Out1 : Outport
  wires:
  Switch2/1 -> Out1/1, soc1/1
  In2/1 -> Sum1/2
  In1/1 -> Sum1/1, Sum/1
  Logical Operator19/1 -> Switch2/2
  Relational Operator3/1 -> Logical Operator19/2
  Type58/1 -> Relational Operator3/2
  Relational Operator2/1 -> Logical Operator19/1
  Type57/1 -> Relational Operator2/2
  Sum/1 -> Switch2/1
  Dot Product2/1 -> Sum/2
  Divide26/1 -> Dot Product2/1
  Type54/1 -> Divide26/2
  Sum1/1 -> Divide26/1
  Clock2/1 -> Sum2/1, Relational Operator2/1, Relational Operator3/1
  Type1/1 -> Sum2/2
  Sum2/1 -> Dot Product2/2

== system Energy_Cost/Battery/Subsystem21 ==
  In1 : Inport
  In2 : Inport  Port=2
  Clock2 : Clock
  Divide26 : Product  Inputs=*/
  Dot Product2 : DotProduct  InputSameDT=on  OutDataTypeStr=Inherit: Inherit via internal rule
  Logical Operator19 : Logic  AllPortsSameDT=off  OutDataTypeStr=boolean
  Relational Operator2 : RelationalOperator  RndMeth=Nearest  InputSameDT=on
  Relational Operator3 : RelationalOperator  Operator=<  RndMeth=Nearest  InputSameDT=on
  Sum : Sum  Inputs=|++
  Sum1 : Sum  Inputs=|-+
  Sum2 : Sum  Inputs=|+-
  Switch2 : Switch  Criteria=u2 > Threshold
  Type1 : Constant  Value=21
  Type54 : Constant
  Type57 : Constant  Value=21
  Type58 : Constant  Value=22
  soc1 : Scope
  Out1 : Outport
  wires:
  Sum2/1 -> Dot Product2/2
  Type1/1 -> Sum2/2
  Clock2/1 -> Relational Operator3/1, Relational Operator2/1, Sum2/1
  Sum1/1 -> Divide26/1
  Type54/1 -> Divide26/2
  Divide26/1 -> Dot Product2/1
  Dot Product2/1 -> Sum/2
  Sum/1 -> Switch2/1
  Type57/1 -> Relational Operator2/2
  Relational Operator2/1 -> Logical Operator19/1
  Type58/1 -> Relational Operator3/2
  Relational Operator3/1 -> Logical Operator19/2
  Logical Operator19/1 -> Switch2/2
  In1/1 -> Sum/1, Sum1/1
  In2/1 -> Sum1/2
  Switch2/1 -> soc1/1, Out1/1

== system Energy_Cost/Battery/Subsystem22 ==
  In1 : Inport
  In2 : Inport  Port=2
  Clock2 : Clock
  Divide26 : Product  Inputs=*/
  Dot Product2 : DotProduct  InputSameDT=on  OutDataTypeStr=Inherit: Inherit via internal rule
  Logical Operator19 : Logic  AllPortsSameDT=off  OutDataTypeStr=boolean
  Relational Operator2 : RelationalOperator  RndMeth=Nearest  InputSameDT=on
  Relational Operator3 : RelationalOperator  Operator=<  RndMeth=Nearest  InputSameDT=on
  Sum : Sum  Inputs=|++
  Sum1 : Sum  Inputs=|-+
  Sum2 : Sum  Inputs=|+-
  Switch2 : Switch  Criteria=u2 > Threshold
  Type1 : Constant  Value=22
  Type54 : Constant
  Type57 : Constant  Value=22
  Type58 : Constant  Value=23
  soc1 : Scope
  Out1 : Outport
  wires:
  Switch2/1 -> Out1/1, soc1/1
  In2/1 -> Sum1/2
  In1/1 -> Sum1/1, Sum/1
  Logical Operator19/1 -> Switch2/2
  Relational Operator3/1 -> Logical Operator19/2
  Type58/1 -> Relational Operator3/2
  Relational Operator2/1 -> Logical Operator19/1
  Type57/1 -> Relational Operator2/2
  Sum/1 -> Switch2/1
  Dot Product2/1 -> Sum/2
  Divide26/1 -> Dot Product2/1
  Type54/1 -> Divide26/2
  Sum1/1 -> Divide26/1
  Clock2/1 -> Sum2/1, Relational Operator2/1, Relational Operator3/1
  Type1/1 -> Sum2/2
  Sum2/1 -> Dot Product2/2

== system Energy_Cost/Battery/Subsystem23 ==
  In1 : Inport
  In2 : Inport  Port=2
  Clock2 : Clock
  Divide26 : Product  Inputs=*/
  Dot Product2 : DotProduct  InputSameDT=on  OutDataTypeStr=Inherit: Inherit via internal rule
  Logical Operator19 : Logic  AllPortsSameDT=off  OutDataTypeStr=boolean
  Relational Operator2 : RelationalOperator  RndMeth=Nearest  InputSameDT=on
  Relational Operator3 : RelationalOperator  Operator=<  RndMeth=Nearest  InputSameDT=on
  Sum : Sum  Inputs=|++
  Sum1 : Sum  Inputs=|-+
  Sum2 : Sum  Inputs=|+-
  Switch2 : Switch  Criteria=u2 > Threshold
  Type1 : Constant  Value=23
  Type54 : Constant
  Type57 : Constant  Value=23
  Type58 : Constant  Value=24
  soc1 : Scope
  Out1 : Outport
  wires:
  Sum2/1 -> Dot Product2/2
  Type1/1 -> Sum2/2
  Clock2/1 -> Relational Operator3/1, Relational Operator2/1, Sum2/1
  Sum1/1 -> Divide26/1
  Type54/1 -> Divide26/2
  Divide26/1 -> Dot Product2/1
  Dot Product2/1 -> Sum/2
  Sum/1 -> Switch2/1
  Type57/1 -> Relational Operator2/2
  Relational Operator2/1 -> Logical Operator19/1
  Type58/1 -> Relational Operator3/2
  Relational Operator3/1 -> Logical Operator19/2
  Logical Operator19/1 -> Switch2/2
  In1/1 -> Sum/1, Sum1/1
  In2/1 -> Sum1/2
  Switch2/1 -> soc1/1, Out1/1

== system Energy_Cost/Battery/Subsystem3 ==
  In1 : Inport
  In2 : Inport  Port=2
  Clock2 : Clock
  Divide26 : Product  Inputs=*/
  Dot Product2 : DotProduct  InputSameDT=on  OutDataTypeStr=Inherit: Inherit via internal rule
  Logical Operator19 : Logic  AllPortsSameDT=off  OutDataTypeStr=boolean
  Relational Operator2 : RelationalOperator  RndMeth=Nearest  InputSameDT=on
  Relational Operator3 : RelationalOperator  Operator=<  RndMeth=Nearest  InputSameDT=on
  Sum : Sum  Inputs=|++
  Sum1 : Sum  Inputs=|-+
  Sum2 : Sum  Inputs=|+-
  Switch2 : Switch  Criteria=u2 > Threshold
  Type1 : Constant  Value=3
  Type54 : Constant
  Type57 : Constant  Value=3
  Type58 : Constant  Value=4
  soc1 : Scope
  Out1 : Outport
  wires:
  Switch2/1 -> Out1/1, soc1/1
  In2/1 -> Sum1/2
  In1/1 -> Sum1/1, Sum/1
  Logical Operator19/1 -> Switch2/2
  Relational Operator3/1 -> Logical Operator19/2
  Type58/1 -> Relational Operator3/2
  Relational Operator2/1 -> Logical Operator19/1
  Type57/1 -> Relational Operator2/2
  Sum/1 -> Switch2/1
  Dot Product2/1 -> Sum/2
  Divide26/1 -> Dot Product2/1
  Type54/1 -> Divide26/2
  Sum1/1 -> Divide26/1
  Clock2/1 -> Sum2/1, Relational Operator2/1, Relational Operator3/1
  Type1/1 -> Sum2/2
  Sum2/1 -> Dot Product2/2

== system Energy_Cost/Battery/Subsystem4 ==
  In1 : Inport
  In2 : Inport  Port=2
  Clock2 : Clock
  Divide26 : Product  Inputs=*/
  Dot Product2 : DotProduct  InputSameDT=on  OutDataTypeStr=Inherit: Inherit via internal rule
  Logical Operator19 : Logic  AllPortsSameDT=off  OutDataTypeStr=boolean
  Relational Operator2 : RelationalOperator  RndMeth=Nearest  InputSameDT=on
  Relational Operator3 : RelationalOperator  Operator=<  RndMeth=Nearest  InputSameDT=on
  Sum : Sum  Inputs=|++
  Sum1 : Sum  Inputs=|-+
  Sum2 : Sum  Inputs=|+-
  Switch2 : Switch  Criteria=u2 > Threshold
  Type1 : Constant  Value=4
  Type54 : Constant
  Type57 : Constant  Value=4
  Type58 : Constant  Value=5
  soc1 : Scope
  Out1 : Outport
  wires:
  Sum2/1 -> Dot Product2/2
  Type1/1 -> Sum2/2
  Clock2/1 -> Relational Operator3/1, Relational Operator2/1, Sum2/1
  Sum1/1 -> Divide26/1
  Type54/1 -> Divide26/2
  Divide26/1 -> Dot Product2/1
  Dot Product2/1 -> Sum/2
  Sum/1 -> Switch2/1
  Type57/1 -> Relational Operator2/2
  Relational Operator2/1 -> Logical Operator19/1
  Type58/1 -> Relational Operator3/2
  Relational Operator3/1 -> Logical Operator19/2
  Logical Operator19/1 -> Switch2/2
  In1/1 -> Sum/1, Sum1/1
  In2/1 -> Sum1/2
  Switch2/1 -> soc1/1, Out1/1

== system Energy_Cost/Battery/Subsystem5 ==
  In1 : Inport
  In2 : Inport  Port=2
  Clock2 : Clock
  Divide26 : Product  Inputs=*/
  Dot Product2 : DotProduct  InputSameDT=on  OutDataTypeStr=Inherit: Inherit via internal rule
  Logical Operator19 : Logic  AllPortsSameDT=off  OutDataTypeStr=boolean
  Relational Operator2 : RelationalOperator  RndMeth=Nearest  InputSameDT=on
  Relational Operator3 : RelationalOperator  Operator=<  RndMeth=Nearest  InputSameDT=on
  Sum : Sum  Inputs=|++
  Sum1 : Sum  Inputs=|-+
  Sum2 : Sum  Inputs=|+-
  Switch2 : Switch  Criteria=u2 > Threshold
  Type1 : Constant  Value=5
  Type54 : Constant
  Type57 : Constant  Value=5
  Type58 : Constant  Value=6
  soc1 : Scope
  Out1 : Outport
  wires:
  Switch2/1 -> Out1/1, soc1/1
  In2/1 -> Sum1/2
  In1/1 -> Sum1/1, Sum/1
  Logical Operator19/1 -> Switch2/2
  Relational Operator3/1 -> Logical Operator19/2
  Type58/1 -> Relational Operator3/2
  Relational Operator2/1 -> Logical Operator19/1
  Type57/1 -> Relational Operator2/2
  Sum/1 -> Switch2/1
  Dot Product2/1 -> Sum/2
  Divide26/1 -> Dot Product2/1
  Type54/1 -> Divide26/2
  Sum1/1 -> Divide26/1
  Clock2/1 -> Sum2/1, Relational Operator2/1, Relational Operator3/1
  Type1/1 -> Sum2/2
  Sum2/1 -> Dot Product2/2

== system Energy_Cost/Battery/Subsystem6 ==
  In1 : Inport
  In2 : Inport  Port=2
  Clock2 : Clock
  Divide26 : Product  Inputs=*/
  Dot Product2 : DotProduct  InputSameDT=on  OutDataTypeStr=Inherit: Inherit via internal rule
  Logical Operator19 : Logic  AllPortsSameDT=off  OutDataTypeStr=boolean
  Relational Operator2 : RelationalOperator  RndMeth=Nearest  InputSameDT=on
  Relational Operator3 : RelationalOperator  Operator=<  RndMeth=Nearest  InputSameDT=on
  Sum : Sum  Inputs=|++
  Sum1 : Sum  Inputs=|-+
  Sum2 : Sum  Inputs=|+-
  Switch2 : Switch  Criteria=u2 > Threshold
  Type1 : Constant  Value=6
  Type54 : Constant
  Type57 : Constant  Value=6
  Type58 : Constant  Value=7
  soc1 : Scope
  Out1 : Outport
  wires:
  Sum2/1 -> Dot Product2/2
  Type1/1 -> Sum2/2
  Clock2/1 -> Relational Operator3/1, Relational Operator2/1, Sum2/1
  Sum1/1 -> Divide26/1
  Type54/1 -> Divide26/2
  Divide26/1 -> Dot Product2/1
  Dot Product2/1 -> Sum/2
  Sum/1 -> Switch2/1
  Type57/1 -> Relational Operator2/2
  Relational Operator2/1 -> Logical Operator19/1
  Type58/1 -> Relational Operator3/2
  Relational Operator3/1 -> Logical Operator19/2
  Logical Operator19/1 -> Switch2/2
  In1/1 -> Sum/1, Sum1/1
  In2/1 -> Sum1/2
  Switch2/1 -> soc1/1, Out1/1

== system Energy_Cost/Battery/Subsystem7 ==
  In1 : Inport
  In2 : Inport  Port=2
  Clock2 : Clock
  Divide26 : Product  Inputs=*/
  Dot Product2 : DotProduct  InputSameDT=on  OutDataTypeStr=Inherit: Inherit via internal rule
  Logical Operator19 : Logic  AllPortsSameDT=off  OutDataTypeStr=boolean
  Relational Operator2 : RelationalOperator  RndMeth=Nearest  InputSameDT=on
  Relational Operator3 : RelationalOperator  Operator=<  RndMeth=Nearest  InputSameDT=on
  Sum : Sum  Inputs=|++
  Sum1 : Sum  Inputs=|-+
  Sum2 : Sum  Inputs=|+-
  Switch2 : Switch  Criteria=u2 > Threshold
  Type1 : Constant  Value=7
  Type54 : Constant
  Type57 : Constant  Value=7
  Type58 : Constant  Value=8
  soc1 : Scope
  Out1 : Outport
  wires:
  Switch2/1 -> Out1/1, soc1/1
  In2/1 -> Sum1/2
  In1/1 -> Sum1/1, Sum/1
  Logical Operator19/1 -> Switch2/2
  Relational Operator3/1 -> Logical Operator19/2
  Type58/1 -> Relational Operator3/2
  Relational Operator2/1 -> Logical Operator19/1
  Type57/1 -> Relational Operator2/2
  Sum/1 -> Switch2/1
  Dot Product2/1 -> Sum/2
  Divide26/1 -> Dot Product2/1
  Type54/1 -> Divide26/2
  Sum1/1 -> Divide26/1
  Clock2/1 -> Sum2/1, Relational Operator2/1, Relational Operator3/1
  Type1/1 -> Sum2/2
  Sum2/1 -> Dot Product2/2

== system Energy_Cost/Battery/Subsystem8 ==
  In1 : Inport
  In2 : Inport  Port=2
  Clock2 : Clock
  Divide26 : Product  Inputs=*/
  Dot Product2 : DotProduct  InputSameDT=on  OutDataTypeStr=Inherit: Inherit via internal rule
  Logical Operator19 : Logic  AllPortsSameDT=off  OutDataTypeStr=boolean
  Relational Operator2 : RelationalOperator  RndMeth=Nearest  InputSameDT=on
  Relational Operator3 : RelationalOperator  Operator=<  RndMeth=Nearest  InputSameDT=on
  Sum : Sum  Inputs=|++
  Sum1 : Sum  Inputs=|-+
  Sum2 : Sum  Inputs=|+-
  Switch2 : Switch  Criteria=u2 > Threshold
  Type1 : Constant  Value=8
  Type54 : Constant
  Type57 : Constant  Value=8
  Type58 : Constant  Value=9
  soc1 : Scope
  Out1 : Outport
  wires:
  Sum2/1 -> Dot Product2/2
  Type1/1 -> Sum2/2
  Clock2/1 -> Relational Operator3/1, Relational Operator2/1, Sum2/1
  Sum1/1 -> Divide26/1
  Type54/1 -> Divide26/2
  Divide26/1 -> Dot Product2/1
  Dot Product2/1 -> Sum/2
  Sum/1 -> Switch2/1
  Type57/1 -> Relational Operator2/2
  Relational Operator2/1 -> Logical Operator19/1
  Type58/1 -> Relational Operator3/2
  Relational Operator3/1 -> Logical Operator19/2
  Logical Operator19/1 -> Switch2/2
  In1/1 -> Sum/1, Sum1/1
  In2/1 -> Sum1/2
  Switch2/1 -> soc1/1, Out1/1

== system Energy_Cost/Battery/Subsystem9 ==
  In1 : Inport
  In2 : Inport  Port=2
  Clock2 : Clock
  Divide26 : Product  Inputs=*/
  Dot Product2 : DotProduct  InputSameDT=on  OutDataTypeStr=Inherit: Inherit via internal rule
  Logical Operator19 : Logic  AllPortsSameDT=off  OutDataTypeStr=boolean
  Relational Operator2 : RelationalOperator  RndMeth=Nearest  InputSameDT=on
  Relational Operator3 : RelationalOperator  Operator=<  RndMeth=Nearest  InputSameDT=on
  Sum : Sum  Inputs=|++
  Sum1 : Sum  Inputs=|-+
  Sum2 : Sum  Inputs=|+-
  Switch2 : Switch  Criteria=u2 > Threshold
  Type1 : Constant  Value=9
  Type54 : Constant
  Type57 : Constant  Value=9
  Type58 : Constant  Value=10
  soc1 : Scope
  Out1 : Outport
  wires:
  Switch2/1 -> Out1/1, soc1/1
  In2/1 -> Sum1/2
  In1/1 -> Sum1/1, Sum/1
  Logical Operator19/1 -> Switch2/2
  Relational Operator3/1 -> Logical Operator19/2
  Type58/1 -> Relational Operator3/2
  Relational Operator2/1 -> Logical Operator19/1
  Type57/1 -> Relational Operator2/2
  Sum/1 -> Switch2/1
  Dot Product2/1 -> Sum/2
  Divide26/1 -> Dot Product2/1
  Type54/1 -> Divide26/2
  Sum1/1 -> Divide26/1
  Clock2/1 -> Sum2/1, Relational Operator2/1, Relational Operator3/1
  Type1/1 -> Sum2/2
  Sum2/1 -> Dot Product2/2

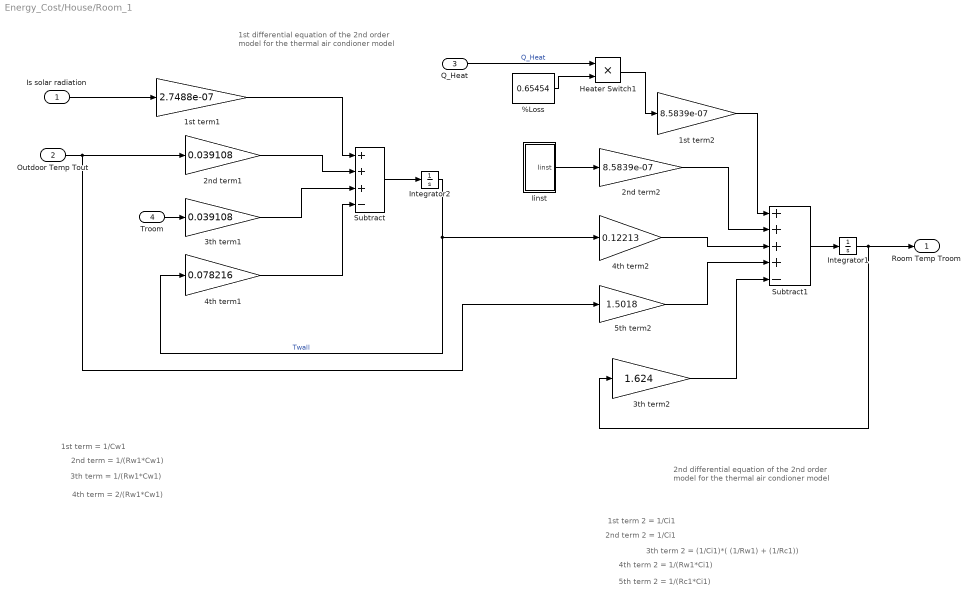
== system Energy_Cost/House/Room_1 ==
  note: 1st differential equation of the 2nd order
      | model for the thermal air condioner model
  note: 2nd differential equation of the 2nd order
      | model for the thermal air condioner model
  note: 1st term = 1/Cw1
  note: 2nd term = 1/(Rw1*Cw1)
  note: 3th term = 1/(Rw1*Cw1)
  note: 4th term = 2/(Rw1*Cw1)
  note: 1st term 2 = 1/Ci1
  note: 2nd term 2 = 1/Ci1
  note: 3th term 2 = (1/Ci1)*( (1/Rw1) + (1/Rc1))
  note: 4th term 2 = 1/(Rw1*Ci1)
  note: 5th term 2 = 1/(Rc1*Ci1)
  Is solar radiation : Inport
  Outdoor Temp Tout : Inport  Port=2
  Q_Heat : Inport  Port=3
  Troom : Inport  Port=4
  %Loss : Constant  Value=0.65454
  1st term1 : Gain  Gain=2.7488e-07
  1st term2 : Gain  Gain=8.5839e-07
  2nd term1 : Gain  Gain=0.039108
  2nd term2 : Gain  Gain=8.5839e-07
  3th term1 : Gain  Gain=0.039108
  3th term2 : Gain  Gain=1.624
  4th term1 : Gain  Gain=0.078216
  4th term2 : Gain  Gain=0.12213
  5th term2 : Gain  Gain=1.5018
  Heater Switch1 : Product  RndMeth=Zero
  Iinst : Subsystem
  Integrator1 : Integrator  InitialCondition=21
  Integrator2 : Integrator  InitialCondition=21
  Subtract : Sum  Inputs=+++-
  Subtract1 : Sum  Inputs=++++-
  Room Temp Troom : Outport  InitialOutput=0
  wires:
  2nd term1/1 -> Subtract/2
  4th term1/1 -> Subtract/4
  Subtract/1 -> Integrator2/1
  Integrator2/1 -> 4th term1/1, 4th term2/1  "Twall"
  Integrator1/1 -> 3th term2/1, Room Temp Troom/1
  Subtract1/1 -> Integrator1/1
  Outdoor Temp Tout/1 -> 2nd term1/1, 5th term2/1
  Troom/1 -> 3th term1/1
  3th term1/1 -> Subtract/3
  1st term1/1 -> Subtract/1
  2nd term2/1 -> Subtract1/2
  Iinst/1(Iinst) -> 2nd term2/1
  Is solar radiation/1 -> 1st term1/1
  4th term2/1 -> Subtract1/3
  5th term2/1 -> Subtract1/4
  3th term2/1 -> Subtract1/5
  Q_Heat/1 -> Heater Switch1/1  "Q_Heat"
  %Loss/1 -> Heater Switch1/2
  1st term2/1 -> Subtract1/1
  Heater Switch1/1 -> 1st term2/1
